simulink model "Copy_of_AutoEncoderPredictSim"  (R2020b)
settings: Solver=VariableStepAuto  StartTime=0.0  StopTime=ts2.Length  RelTol=1e-3
undefined symbols (not defined in the file): threshold
libraries: simulink x1, dspmtrx3 x1, dspstat3 x1, deeplib x1
settings Model: Creator=Alia  LastModifiedBy=Alia

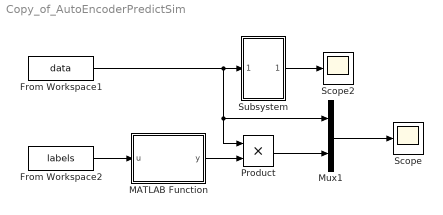
== system Copy_of_AutoEncoderPredictSim ==
  From Workspace1 : FromWorkspace  VariableName=data
  From Workspace2 : FromWorkspace  VariableName=labels
  MATLAB Function : MATLAB Function  TreatAsAtomicUnit=on
  Mux1 : Mux  Inputs=2
  Product : Product
  Scope : Scope
  Scope2 : Scope
  Subsystem : Subsystem  mask{BufferLength=40, NetworkFilePath=C:\Users\Alia\Desktop\BA Anomaly Detection\Matlab generation\ALL Data\net.mat, InputDataFormats={ '', '' }}
      mask prompts: BufferLength "dspshared:blkprm_prompts:OutputBufferSize"; NetworkFilePath "deep_blocks:common:FilePath"; InputDataFormats "deep_blocks:predict:InputDataFormats"
      mask help: Buffer overload value must be equal to 1-BufferSize
      mask TypeOptions BufferLength:
      | Buffer/N | Delay/DelayLength | Compare
      | To Constant/const
      mask TypeOptions NetworkFilePath: Predict1/NetworkFilePath | Predict1/NetworkFunction
      mask TypeOptions InputDataFormats: Predict1/InputDataFormats
      mask DialogControl BufferLength Prompt: Output buffer size (per channel):
      mask DialogControl NetworkFilePath Prompt: File path:
      mask DialogControl Control2 Prompt: Browse
      mask DialogControl InputDataFormats Prompt: Input data formats:
  wires:
  Mux1/1 -> Scope/1
  From Workspace2/1 -> MATLAB Function/1(u)
  From Workspace1/1 -> Mux1/1, Product/1, Subsystem/1(In1)
  MATLAB Function/1(y) -> Product/2
  Product/1 -> Mux1/2
  Subsystem/1(Out1) -> Scope2/1

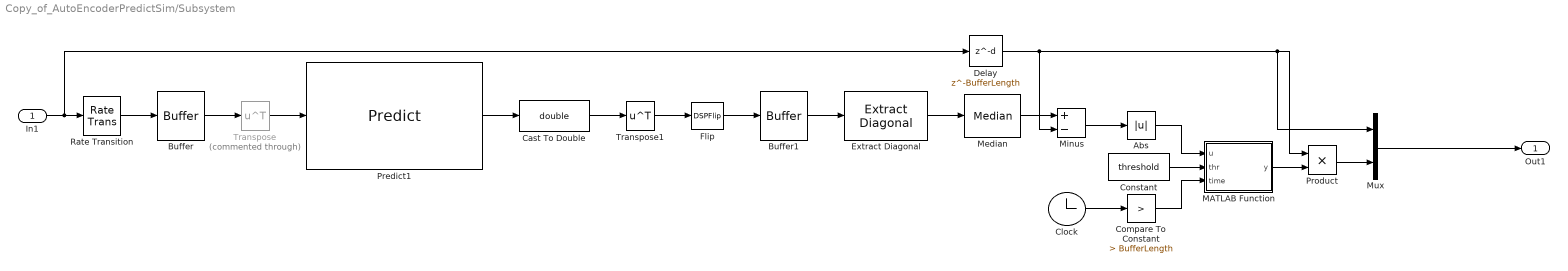
== system Copy_of_AutoEncoderPredictSim/Subsystem ==
  In1 : Inport
  Abs : Abs
  Buffer : Buffer  N=BufferLength  V=BufferLength-1  OutputFrames=off
  Buffer1 : Buffer  N=BufferLength  V=BufferLength-1  OutputFrames=off
  Cast To Double : DataTypeConversion  OutDataTypeStr=double
  Clock : Clock
  Compare To Constant : simulink/Logic and Bit Operations/Compare To Constant  relop=>  const=BufferLength  OutDataTypeStr=boolean
  Constant : Constant  Value=threshold
  Delay : Delay  DelayLength=BufferLength
  Extract Diagonal : dspmtrx3/Extract Diagonal
      settings: SourceProductBaseCode=DS
  Flip : DSPFlip
  MATLAB Function : MATLAB Function  TreatAsAtomicUnit=on
  Median : dspstat3/Median  sortAlg=Quick sort  directionMode=Each column  dimension=1  roundingMode=Floor  overflowMode=off  accumDataTypeStr=Inherit: Same as product output  accumLastDataTypeStr=Inherit: Same as product output  outputDataTypeStr=Inherit: Same as accumulator  outputMin=[]  outputMax=[]  outputLastDataTypeStr=Inherit: Same as accumulator
      settings: SourceProductBaseCode=DS  allowOverrides=off
  Minus : Sum  Inputs=+-
  Mux : Mux  Inputs=2
  Predict1 : deeplib/Predict  Network=Network from MAT-file  NetworkFunction=C:\Users\Alia\Desktop\BA Anomaly Detection\Matlab generation\ALL Data\net.mat  NetworkFilePath=C:\Users\Alia\Desktop\BA Anomaly Detection\Matlab generation\ALL Data\net.mat  MiniBatchSize=128  InputDataFormats={ '', '' }  Predictions=on  Activations={}  ForceInterpretedSim=off  EnableDLNetwork=off
      settings: SourceProductBaseCode=NN
  Product : Product
  Rate Transition : RateTransition  OutPortSampleTime=1
  Transpose : Math  Commented=through  Operator=transpose  SaturateOnIntegerOverflow=on
  Transpose1 : Math  Operator=transpose  SaturateOnIntegerOverflow=on
  Out1 : Outport
  wires:
  Mux/1 -> Out1/1
  Transpose1/1 -> Flip/1
  Extract Diagonal/1 -> Median/1
  In1/1 -> Delay/1, Rate Transition/1
  Buffer1/1 -> Extract Diagonal/1
  MATLAB Function/1(y) -> Product/2
  Clock/1 -> Compare To Constant/1
  Abs/1 -> MATLAB Function/1(u)
  Flip/1 -> Buffer1/1
  Predict1/1 -> Cast To Double/1
  Cast To Double/1 -> Transpose1/1
  Rate Transition/1 -> Buffer/1
  Median/1 -> Minus/1
  Constant/1 -> MATLAB Function/2(thr)
  Product/1 -> Mux/2
  Minus/1 -> Abs/1
  Compare To Constant/1 -> MATLAB Function/3(time)
  Buffer/1 -> Transpose/1
  Transpose/1 -> Predict1/1
  Delay/1 -> Mux/1, Product/1, Minus/2

== matlab function Copy_of_AutoEncoderPredictSim/MATLAB Function ==
  data: u input; y output
function y = fcn(u)
y = NaN;
if u == 1
    y = 1;
end

== matlab function Copy_of_AutoEncoderPredictSim/Subsystem/MATLAB Function ==
  data: u input; y output; thr input; time input
function y = fcn(u,thr, time)
y = NaN;
if time == 1
    if u > thr
    y = 1;
    end
end
